simulink model "Dual_Clutch_Trans_SDO_org"  (Simulink 10.0)
settings: Solver=ode1  StartTime=0.0  StopTime=15  MaxStep=0.1  RelTol=1e-3  EnableMultiTasking=on
PreLoadFcn:
  | load UrbanCycle1;
  | load UrbanCycle2;
  | load UrbanCycle3;
  | load UrbanCycle4;
  | load UrbanCycle5;
  | load UrbanCycle6;
  | load UrbanCycle7;
  | load UrbanCycle8;
  | Shift_Gear_Delay = 50;
  | Ratio_Time_Const = 0.1;
  | Drive_Cycle_Num = 7;
  | load RefRPMData;
PostLoadFcn:
  | warning off Simulink:SampleTime:TsPropEnabOutputsChangeNotAligned;
  | warning off Simulink:blocks:MatchingFromNotFound
  | warning off Simulink:blocks:MatchingGotoNotFound
  | warning off Simulink:Engine:OutputNotConnected
  | warning off Simulink:Engine:LineWithoutDst
  | warning off Simulink:Engine:UINotUpdatedDuringRapidAccelSim
  | warning off Simulink:Commands:SetParamLinkChangeWarn
  | warning off Simulink:Engine:SaveWithParameterizedLinks_Warning
undefined symbols (not defined in the file): DCT_Param, Downshift_Speeds, sigbuilder_block, Upshift_Speeds
libraries: fl_lib x5, nesl_utility x4, simulink x3, sdl_lib x2, DCT_Vehicle_Dynamics_Lib x2, Engine_Lib x1
(part 2 of 2)

== stateflow chart Transmission Controller/Shift state/Chart ==
  settings: sampleTime=0.01
  state GearState [parallel]
    settings: executionOrder=1
    state G1
      en: GearState=1;
      en:C1=1;C2=0;
      NGsf=2;
    state G3
      en: GearState=3;
      du:[SpdThr]=calc(3,pedal,speed);
      (history)
      state NGlow
        en: NGsf=2;
      state NGhigh
        en: NGsf=4;
      (default) -> GearState.G3.NGlow
      GearState.G3.NGlow -> GearState.G3.NGhigh : [SpdThr<0 &&...
          | GearState==3]
      GearState.G3.NGhigh -> GearState.G3.NGlow : [SpdThr>=0 &&...
          | GearState==3]
    state G2
      en: GearState=2;
      du:[SpdThr]=calc(2,pedal,speed);
      (history)
      state NGlow
        en: NGsf=1;
      state NGhigh
        en: NGsf=3;
      (default) -> GearState.G2.NGlow
      GearState.G2.NGlow -> GearState.G2.NGhigh : [SpdThr<0 &&...
          |  GearState==2]
      GearState.G2.NGhigh -> GearState.G2.NGlow : [SpdThr>=0 &&...
          |  GearState==2]
    state Launch
      en: GearState=0.5;
      en:C1=0;C2=0;
      NGsf=1;
    state G5
      en:GearState=5;
      du:[SpdThr]=calc(5,pedal,speed);
      (history)
      state NGlow
        en: NGsf=4;
      state NGhigh
        en: NGsf=6;
      (default) -> GearState.G5.NGlow
      GearState.G5.NGlow -> GearState.G5.NGhigh : [SpdThr<0 &&...
          | GearState==5]
      GearState.G5.NGhigh -> GearState.G5.NGlow : [SpdThr>=0 &&...
          | GearState==5]
    state G6
      en:GearState=6;
      NGsf=5;
    state G4
      en:GearState=4;
      du:[SpdThr]=calc(4,pedal,speed);
      (history)
      state NGlow
        en: NGsf=3;
      state NGhigh
        en: NGsf=5;
      (default) -> GearState.G4.NGlow
      GearState.G4.NGlow -> GearState.G4.NGhigh : [SpdThr<0 &&...
          | GearState==4]
      GearState.G4.NGhigh -> GearState.G4.NGlow : [SpdThr>=0 &&...
          | GearState==4]
    G1 -> G2 [order 1] : Up
    Launch -> G1 : [abs(S1)<10 && RPM>850]
        | {clutchControl=1;}
    G2 -> G3 [order 1] : Up
    G3 -> G2 [order 2] : Down
    G1 -> Launch [order 2] : [RPM<800]
        | {clutchControl=-1;}
    G2 -> G1 [order 2] : Down
    (default) -> Launch
    G3 -> G4 [order 1] : Up
    G4 -> G3 [order 2] : Down
    G4 -> G5 [order 1] : Up
    G5 -> G6 [order 1] : Up
    G6 -> G5 : Down
    G5 -> G4 [order 2] : Down
  state SelectionState [parallel]
    du:[up_th]=calc_up(GearState,pedal);
    du:[down_th]=calc_down(GearState,pedal);
    settings: executionOrder=2
    state SteadyState
      en:clutchControl=0;
    state preDownShifting
    state preUpShifting
    state UpShifting
      en: GearState=GearState+0.5;
      en:[C1,C2] = clutchstates...
      (GearState,clutchControl)
    state DownShifting
      en: GearState=GearState-0.5;
      en:[C1,C2] = clutchstates...
      (GearState,clutchControl)
    (default) -> SteadyState
    SteadyState -> (junction 60) [order 1] : [speed < down_th && ...
        | GearState >1]
        | {clutchControl=-1;}
    SteadyState -> (junction 61) [order 2] : [speed > up_th &&...
        | GearState <=5 && ...
        | floor(GearState) == GearState]
        | {clutchControl=1;}
    (junction 60) -> preDownShifting
    (junction 61) -> preUpShifting
    (junction 62) -> SteadyState
    (junction 64) -> SteadyState
    (junction 63) -> SteadyState
    preDownShifting -> (junction 62) [order 2] : [speed >= down_th]
    preUpShifting -> (junction 63) [order 2] : [speed <= up_th]
    preUpShifting -> UpShifting [order 1] : after(0.5,sec)
        | [speed>up_th]
    preDownShifting -> DownShifting [order 1] : after(0.5,sec)
        | [speed < down_th-2]
    DownShifting -> (junction 64) : [shiftComplete ==1]
        | {GearState.Down;}
    UpShifting -> (junction 64) : [shiftComplete==1]
        | {GearState.Up;}
  state up_th = calc_up(gear,pedal) [function]
  state down_th = calc_down(gear,pedal) [function]
  state SpdThr = calc(gear,pedal,speed) [function]
  data: gear function_input double; pedal function_input double; up_th function_output double; gear function_input double; pedal function_input double; down_th function_output double; gear function_input double; pedal function_input double; SpdThr function_output double; speed function_input double; gear function_input double; updown function_input double; cl1 function_output double; cl2 function_output double; GearState output double; S1 input double; shiftComplete input double; speed input double; pedal input double; up_th output double; down_th output double; RPM input double; NGsf output double; C1 output double; C2 output double; clutchControl local double; SpdThr local double
  events: Up local EITHER_EDGE_EVENT; Down local EITHER_EDGE_EVENT
  function [cl1,cl2] = clutchstates(gear,updown):
    | function [cl1,cl2] = clutchstates(gear,updown) 
    | if (((gear==1.5)||(gear==3.5)||(gear==5.5))&&(updown==1) || ((gear==2.5)||(gear==4.5))&&(updown==-1))
    |     cl1 = 0;
    |     cl2 = 1;
    | else%if((gear==1.5)||(gear==3.5))&&(updown==-1) || ((gear==2.5)||(gear==4.5))&&(updown==1)
    | 	cl1 = 1;
    |     cl2 = 0;
    | end
